simulink model "Modelpa"  (Simulink 8.5)
settings: Solver=ode45  StartTime=0.0  StopTime=0.1  RelTol=1e-3
values from neighbouring files (symbols this model uses):
  u11pa = U1_(j,i+1)    [EDMC.m]    (also in EDMC_with_Constraint.m; Vri.m)
  u11per = U1per(j,i+1)    [EDMC.m]    (also in EDMC_with_Constraint.m; Vri.m)
  u1pa = U1_(j,i+1)    [EDMC.m]    (also in EDMC_with_Constraint.m; Vri.m)
  u22pa = U2_(j,i+1)    [EDMC.m]    (also in EDMC_with_Constraint.m; Vri.m)
  u22per = U2per(j,i+1)    [EDMC.m]    (also in EDMC_with_Constraint.m; Vri.m)
  u2pa = U2_(j,i+1)    [EDMC.m]    (also in EDMC_with_Constraint.m; Vri.m)
  x011pa = x1pa1(end)    [EDMC.m]    (also in EDMC_with_Constraint.m; Vri.m)
  x011per = x1per1(end)    [EDMC.m]    (also in EDMC_with_Constraint.m; Vri.m)
  x012pa = x1pa2(end)    [EDMC.m]    (also in EDMC_with_Constraint.m; Vri.m)
  x012per = x1per2(end)    [EDMC.m]    (also in EDMC_with_Constraint.m; Vri.m)
  x01pa = x1pa(end)    [EDMC.m]    (also in EDMC_with_Constraint.m; Vri.m)
  x021pa = x2pa1(end)    [EDMC.m]    (also in EDMC_with_Constraint.m; Vri.m)
  x021per = x2per1(end)    [EDMC.m]    (also in EDMC_with_Constraint.m; Vri.m)
  x022pa = x2pa2(end)    [EDMC.m]    (also in EDMC_with_Constraint.m; Vri.m)
  x022per = x2per2(end)    [EDMC.m]    (also in EDMC_with_Constraint.m; Vri.m)
  x02pa = x2pa(end)    [EDMC.m]    (also in EDMC_with_Constraint.m; Vri.m)
settings Model: Creator=Default  LastModifiedBy=Default
settings DataIOCC: SignalLoggingSaveFormat=Dataset
settings OptimizationCC: ExpressionDepthLimit=128
settings DebuggingCC: UnderspecifiedInitializationDetection=Simplified  MergeDetectMultiDrivingBlocksExec=error  FcnCallInpInsideContextMsg=EnableAllAsError  StateNameClashWarn=none
settings GRTTargetCC: CombineOutputUpdateFcns=on  GRTInterface=off

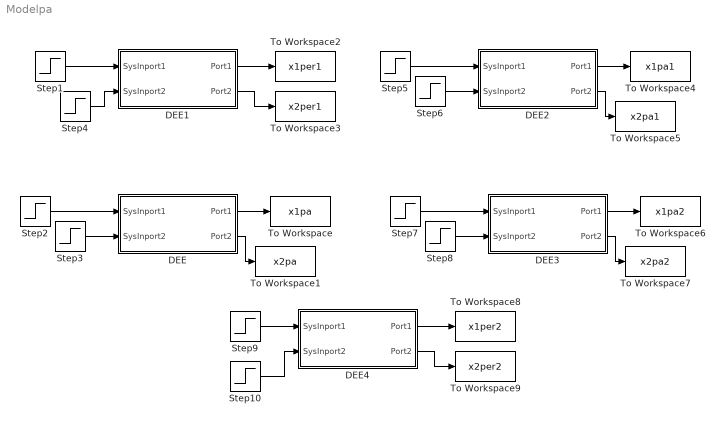
== system Modelpa ==
  DEE : Subsystem  mask(Differential Equation Editor (DEE)){}
      settings: OpenFcn=diffeqed
      mask Display: disp('Differential Equation\n Editor')
  DEE1 : Subsystem  mask(Differential Equation Editor (DEE)){}
      settings: OpenFcn=diffeqed
      mask Display: disp('Differential Equation\n Editor')
  DEE2 : Subsystem  mask(Differential Equation Editor (DEE)){}
      settings: OpenFcn=diffeqed
      mask Display: disp('Differential Equation\n Editor')
  DEE3 : Subsystem  mask(Differential Equation Editor (DEE)){}
      settings: OpenFcn=diffeqed
      mask Display: disp('Differential Equation\n Editor')
  DEE4 : Subsystem  mask(Differential Equation Editor (DEE)){}
      settings: OpenFcn=diffeqed
      mask Display: disp('Differential Equation\n Editor')
  Step1 : Step  Time=0  After=u11per  SampleTime=0
  Step10 : Step  Time=0  After=u22per  SampleTime=0
  Step2 : Step  Time=0  After=u1pa  SampleTime=0
  Step3 : Step  Time=0  After=u2pa  SampleTime=0
  Step{4,6..7,9} (4 alike) : Step  Time=0  After=100  SampleTime=0
  Step5 : Step  Time=0  After=u11pa  SampleTime=0
  Step8 : Step  Time=0  After=u22pa  SampleTime=0
  To Workspace : ToWorkspace  VariableName=x1pa  SampleTime=-1
  To Workspace1 : ToWorkspace  VariableName=x2pa  SampleTime=-1
  To Workspace2 : ToWorkspace  VariableName=x1per1  SampleTime=-1
  To Workspace3 : ToWorkspace  VariableName=x2per1  SampleTime=-1
  To Workspace4 : ToWorkspace  VariableName=x1pa1  SampleTime=-1
  To Workspace5 : ToWorkspace  VariableName=x2pa1  SampleTime=-1
  To Workspace6 : ToWorkspace  VariableName=x1pa2  SampleTime=-1
  To Workspace7 : ToWorkspace  VariableName=x2pa2  SampleTime=-1
  To Workspace8 : ToWorkspace  VariableName=x1per2  SampleTime=-1
  To Workspace9 : ToWorkspace  VariableName=x2per2  SampleTime=-1
  wires:
  Step2/1 -> DEE/1(SysInport1)
  DEE/1(Port1) -> To Workspace/1
  DEE/2(Port2) -> To Workspace1/1
  Step3/1 -> DEE/2(SysInport2)
  Step1/1 -> DEE1/1(SysInport1)
  DEE1/1(Port1) -> To Workspace2/1
  DEE1/2(Port2) -> To Workspace3/1
  Step4/1 -> DEE1/2(SysInport2)
  Step5/1 -> DEE2/1(SysInport1)
  DEE2/1(Port1) -> To Workspace4/1
  DEE2/2(Port2) -> To Workspace5/1
  Step6/1 -> DEE2/2(SysInport2)
  Step7/1 -> DEE3/1(SysInport1)
  DEE3/1(Port1) -> To Workspace6/1
  DEE3/2(Port2) -> To Workspace7/1
  Step8/1 -> DEE3/2(SysInport2)
  Step9/1 -> DEE4/1(SysInport1)
  DEE4/1(Port1) -> To Workspace8/1
  DEE4/2(Port2) -> To Workspace9/1
  Step10/1 -> DEE4/2(SysInport2)

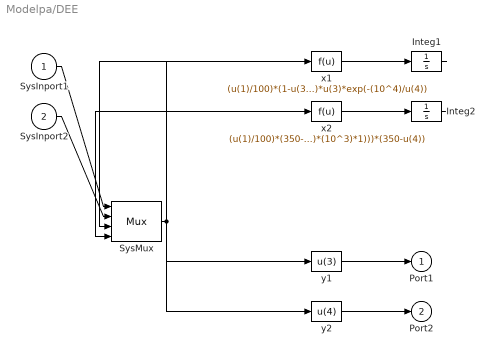
== system Modelpa/DEE ==
  SysInport1 : Inport
  SysInport2 : Inport  Port=2
  Integ1 : Integrator  InitialCondition=x01pa
  Integ2 : Integrator  InitialCondition=x02pa
  SysMux : Mux
  x1 : Fcn  Expr=(u(1)/100)*(1-u(3))-(7.2*10^10)*u(3)*exp(-(10^4)/u(4))
  x2 : Fcn  Expr=(u(1)/100)*(350-u(4))-((-(2*10^5)/(10^3))*(7.2*10^10)*u(3)*exp(-(10^4)/u(4)))+(((10^3)*1)/((10^3)*100))*(u(2))*(1-exp(-(7*10^5)/(u(2)*(10^3)*1)))*(350-u(4))
  y1 : Fcn  Expr=u(3)
  y2 : Fcn  Expr=u(4)
  Port1 : Outport
  Port2 : Outport  Port=2
  wires:
  SysInport1/1 -> SysMux/1
  SysInport2/1 -> SysMux/2
  SysMux/1 -> x1/1, x2/1, y1/1, y2/1
  x1/1 -> Integ1/1
  Integ1/1 -> SysMux/3
  x2/1 -> Integ2/1
  Integ2/1 -> SysMux/4
  y1/1 -> Port1/1
  y2/1 -> Port2/1

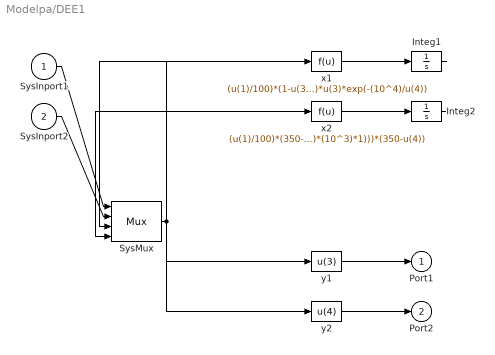
== system Modelpa/DEE1 ==
  SysInport1 : Inport
  SysInport2 : Inport  Port=2
  Integ1 : Integrator  InitialCondition=x011per
  Integ2 : Integrator  InitialCondition=x021per
  SysMux : Mux
  x1 : Fcn  Expr=(u(1)/100)*(1-u(3))-(7.2*10^10)*u(3)*exp(-(10^4)/u(4))
  x2 : Fcn  Expr=(u(1)/100)*(350-u(4))-((-(2*10^5)/(10^3))*(7.2*10^10)*u(3)*exp(-(10^4)/u(4)))+(((10^3)*1)/((10^3)*100))*(u(2))*(1-exp(-(7*10^5)/(u(2)*(10^3)*1)))*(350-u(4))
  y1 : Fcn  Expr=u(3)
  y2 : Fcn  Expr=u(4)
  Port1 : Outport
  Port2 : Outport  Port=2
  wires:
  SysInport1/1 -> SysMux/1
  SysInport2/1 -> SysMux/2
  SysMux/1 -> x1/1, x2/1, y1/1, y2/1
  x1/1 -> Integ1/1
  Integ1/1 -> SysMux/3
  x2/1 -> Integ2/1
  Integ2/1 -> SysMux/4
  y1/1 -> Port1/1
  y2/1 -> Port2/1

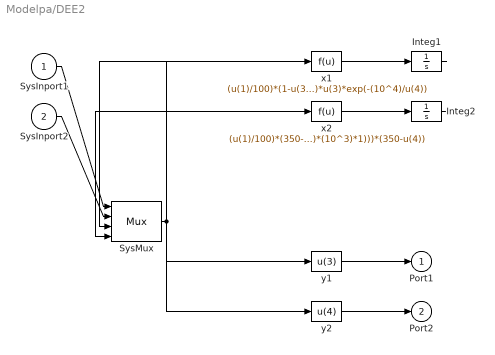
== system Modelpa/DEE2 ==
  SysInport1 : Inport
  SysInport2 : Inport  Port=2
  Integ1 : Integrator  InitialCondition=x011pa
  Integ2 : Integrator  InitialCondition=x021pa
  SysMux : Mux
  x1 : Fcn  Expr=(u(1)/100)*(1-u(3))-(7.2*10^10)*u(3)*exp(-(10^4)/u(4))
  x2 : Fcn  Expr=(u(1)/100)*(350-u(4))-((-(2*10^5)/(10^3))*(7.2*10^10)*u(3)*exp(-(10^4)/u(4)))+(((10^3)*1)/((10^3)*100))*(u(2))*(1-exp(-(7*10^5)/(u(2)*(10^3)*1)))*(350-u(4))
  y1 : Fcn  Expr=u(3)
  y2 : Fcn  Expr=u(4)
  Port1 : Outport
  Port2 : Outport  Port=2
  wires:
  SysInport1/1 -> SysMux/1
  SysInport2/1 -> SysMux/2
  SysMux/1 -> x1/1, x2/1, y1/1, y2/1
  x1/1 -> Integ1/1
  Integ1/1 -> SysMux/3
  x2/1 -> Integ2/1
  Integ2/1 -> SysMux/4
  y1/1 -> Port1/1
  y2/1 -> Port2/1

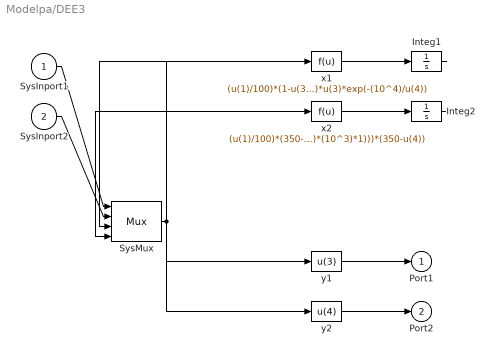
== system Modelpa/DEE3 ==
  SysInport1 : Inport
  SysInport2 : Inport  Port=2
  Integ1 : Integrator  InitialCondition=x012pa
  Integ2 : Integrator  InitialCondition=x022pa
  SysMux : Mux
  x1 : Fcn  Expr=(u(1)/100)*(1-u(3))-(7.2*10^10)*u(3)*exp(-(10^4)/u(4))
  x2 : Fcn  Expr=(u(1)/100)*(350-u(4))-((-(2*10^5)/(10^3))*(7.2*10^10)*u(3)*exp(-(10^4)/u(4)))+(((10^3)*1)/((10^3)*100))*(u(2))*(1-exp(-(7*10^5)/(u(2)*(10^3)*1)))*(350-u(4))
  y1 : Fcn  Expr=u(3)
  y2 : Fcn  Expr=u(4)
  Port1 : Outport
  Port2 : Outport  Port=2
  wires:
  SysInport1/1 -> SysMux/1
  SysInport2/1 -> SysMux/2
  SysMux/1 -> x1/1, x2/1, y1/1, y2/1
  x1/1 -> Integ1/1
  Integ1/1 -> SysMux/3
  x2/1 -> Integ2/1
  Integ2/1 -> SysMux/4
  y1/1 -> Port1/1
  y2/1 -> Port2/1

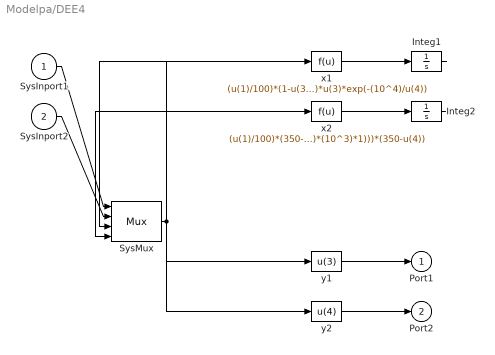
== system Modelpa/DEE4 ==
  SysInport1 : Inport
  SysInport2 : Inport  Port=2
  Integ1 : Integrator  InitialCondition=x012per
  Integ2 : Integrator  InitialCondition=x022per
  SysMux : Mux
  x1 : Fcn  Expr=(u(1)/100)*(1-u(3))-(7.2*10^10)*u(3)*exp(-(10^4)/u(4))
  x2 : Fcn  Expr=(u(1)/100)*(350-u(4))-((-(2*10^5)/(10^3))*(7.2*10^10)*u(3)*exp(-(10^4)/u(4)))+(((10^3)*1)/((10^3)*100))*(u(2))*(1-exp(-(7*10^5)/(u(2)*(10^3)*1)))*(350-u(4))
  y1 : Fcn  Expr=u(3)
  y2 : Fcn  Expr=u(4)
  Port1 : Outport
  Port2 : Outport  Port=2
  wires:
  SysInport1/1 -> SysMux/1
  SysInport2/1 -> SysMux/2
  SysMux/1 -> x1/1, x2/1, y1/1, y2/1
  x1/1 -> Integ1/1
  Integ1/1 -> SysMux/3
  x2/1 -> Integ2/1
  Integ2/1 -> SysMux/4
  y1/1 -> Port1/1
  y2/1 -> Port2/1
